simulink library "findClosestPointOnPath_cl"  (R2018a)
settings: Solver=VariableStepAuto  StartTime=0.0  StopTime=10.0  RelTol=1e-3
undefined symbols (not defined in the file): ctrl
libraries: controllerComponents x3, dspstat3 x1
settings Model: Creator=mitch  LastModifiedBy=mitch

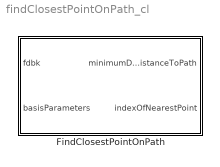
== system findClosestPointOnPath_cl ==
  FindClosestPointOnPath : Subsystem

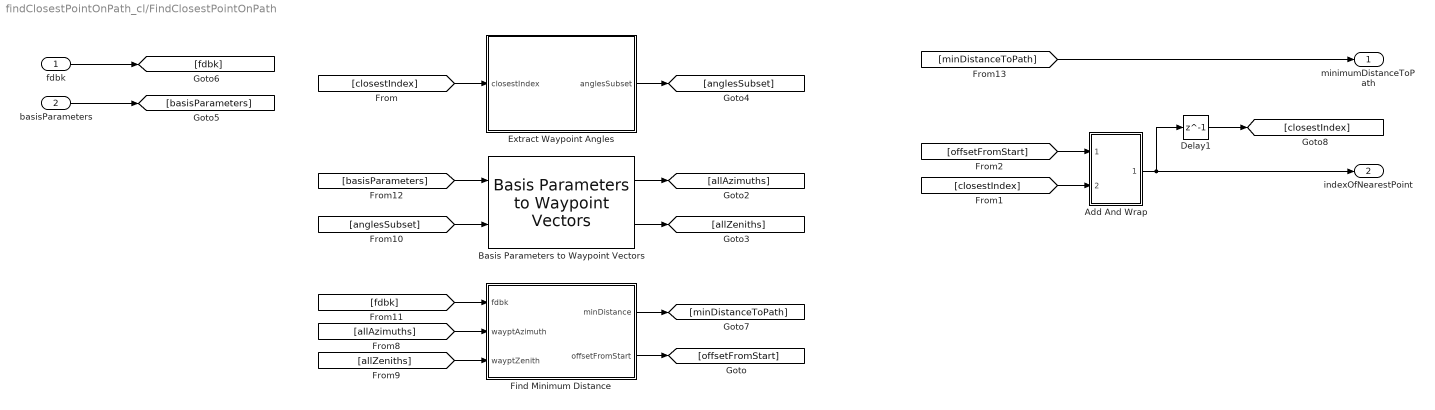
== system findClosestPointOnPath_cl/FindClosestPointOnPath ==
  fdbk : Inport
  basisParameters : Inport  Port=2
  Add And Wrap : Subsystem
  Basis Parameters to Waypoint Vectors : controllerComponents/Basis Parameters to Waypoint Vectors
  Delay1 : Delay  DelayLength=1  InitialCondition=1
  Extract Waypoint Angles : Subsystem
  Find Minimum Distance : Subsystem
  minimumDistanceToPath : Outport
  indexOfNearestPoint : Outport  Port=2
  wires:
  [closestIndex] -> Extract Waypoint Angles/1(closestIndex)
  Basis Parameters to Waypoint Vectors/2 -> [allZeniths]
  Basis Parameters to Waypoint Vectors/1 -> [allAzimuths]
  Extract Waypoint Angles/1(anglesSubset) -> [anglesSubset]
  [anglesSubset] -> Basis Parameters to Waypoint Vectors/2
  basisParameters/1 -> [basisParameters]
  fdbk/1 -> [fdbk]
  [basisParameters] -> Basis Parameters to Waypoint Vectors/1
  [minDistanceToPath] -> minimumDistanceToPath/1
  [fdbk] -> Find Minimum Distance/1(fdbk)
  [allAzimuths] -> Find Minimum Distance/2(wayptAzimuth)
  [allZeniths] -> Find Minimum Distance/3(wayptZenith)
  Find Minimum Distance/1(minDistance) -> [minDistanceToPath]
  Find Minimum Distance/2(offsetFromStart) -> [offsetFromStart]
  [offsetFromStart] -> Add And Wrap/1(offset)
  [closestIndex] -> Add And Wrap/2(startIndex)
  Add And Wrap/1(Out1) -> Delay1/1, indexOfNearestPoint/1
  Delay1/1 -> [closestIndex]

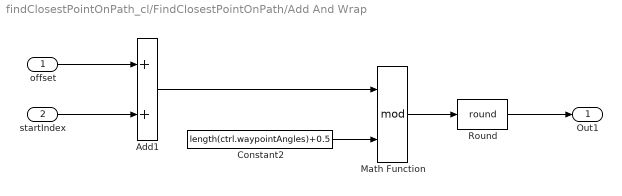
== system findClosestPointOnPath_cl/FindClosestPointOnPath/Add And Wrap ==
  offset : Inport
  startIndex : Inport  Port=2
  Add1 : Sum
  Constant2 : Constant  Value=length(ctrl.waypointAngles)+0.5  SampleTime=-1
  Math Function : Math  Operator=mod  SaturateOnIntegerOverflow=on
  Round : Rounding  Operator=round
  Out1 : Outport
  wires:
  offset/1 -> Add1/1
  startIndex/1 -> Add1/2
  Add1/1 -> Math Function/1
  Constant2/1 -> Math Function/2
  Math Function/1 -> Round/1
  Round/1 -> Out1/1

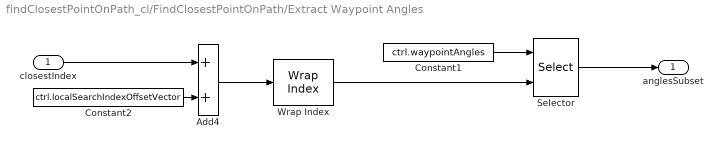
== system findClosestPointOnPath_cl/FindClosestPointOnPath/Extract Waypoint Angles ==
  closestIndex : Inport
  Add4 : Sum
  Constant1 : Constant  Value=ctrl.waypointAngles  SampleTime=-1
  Constant2 : Constant  Value=ctrl.localSearchIndexOffsetVector  SampleTime=-1
  Selector : Selector  InputPortWidth=length(ctrl.waypointAngles)  IndexOptions=Index vector (port)  Indices=[1 3]  OutputSizes=1
  Wrap Index : controllerComponents/Wrap Index
  anglesSubset : Outport
  wires:
  Selector/1 -> anglesSubset/1
  Wrap Index/1 -> Selector/2
  Add4/1 -> Wrap Index/1
  Constant2/1 -> Add4/2
  Constant1/1 -> Selector/1
  closestIndex/1 -> Add4/1

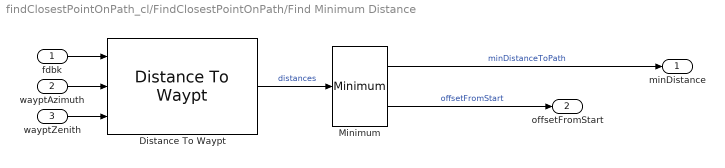
== system findClosestPointOnPath_cl/FindClosestPointOnPath/Find Minimum Distance ==
  fdbk : Inport
  wayptAzimuth : Inport  Port=2
  wayptZenith : Inport  Port=3
  Distance To Waypt : controllerComponents/Distance To Waypt
  Minimum : dspstat3/Minimum  operation=minimum  fcn=Value and Index  indexBase=Zero  operateOver=Entire input  Dimension=1  InputProcessing=Columns as channels (frame based)  reset=None  roiEnable=off  roiType=Rectangles  roiPortion=Entire ROI  roiOutput=Individual statistics for each ROI  roiFlag=off  roundingMode=Floor  overflowMode=off
      settings: SourceProductName=DSP System Toolbox  SourceProductBaseCode=DS
  minDistance : Outport
  offsetFromStart : Outport  Port=2
  wires:
  Distance To Waypt/1 -> Minimum/1  "distances"
  wayptAzimuth/1 -> Distance To Waypt/2
  Minimum/1 -> minDistance/1  "minDistanceToPath"
  wayptZenith/1 -> Distance To Waypt/3
  fdbk/1 -> Distance To Waypt/1
  Minimum/2 -> offsetFromStart/1  "offsetFromStart"
